simulink model "ProjectSimulink_2"  (R2023b)
settings: Solver=VariableStepAuto  StartTime=0.0  StopTime=10.0  RelTol=1e-3
libraries: simulink x1
settings Model: Creator=Davide  LastModifiedBy=Davide

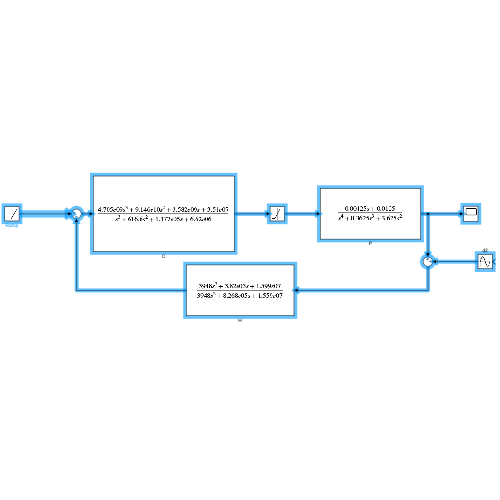
[thumbnail: Simulink's stored preview of the top-level diagram]
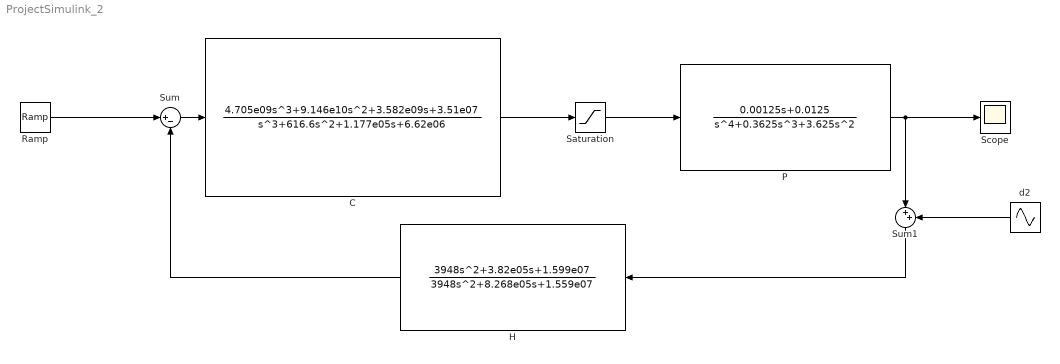
== system ProjectSimulink_2 ==
  C : TransferFcn  Numerator=[4.705e09 9.146e10 3.582e09 3.51e07]  Denominator=[1 616.6 1.177e05 6.62e06]
  H : TransferFcn  Numerator=[3948 3.82e05 1.599e07]  Denominator=[3948 8.268e05 1.559e07]
  P : TransferFcn  Numerator=[0.00125 0.0125]  Denominator=[1 0.3625 3.625 0 0]
  Ramp : simulink/Sources/Ramp  slope=1  start=0  InitialOutput=0
  Saturation : Saturate  UpperLimit=0.01  LowerLimit=-0.01
  Scope : Scope
  Sum : Sum  Inputs=|+-
  Sum1 : Sum  Inputs=|++
  d2 : Sin  TimeSource=Use external signal  Frequency=62.8  SampleTime=0.01
  wires:
  Sum1/1 -> H/1
  P/1 -> Scope/1, Sum1/1
  Sum/1 -> C/1
  C/1 -> Saturation/1
  H/1 -> Sum/2
  Saturation/1 -> P/1
  d2/1 -> Sum1/2
  Ramp/1 -> Sum/1
